simulink model "exercise02"  (R2022a)
settings: Solver=VariableStepAuto  StartTime=0.0  StopTime=10  RelTol=1e-3
settings Model: Creator=ac133867  LastModifiedBy=cunis
settings DebuggingCC: UnconnectedInputMsg=warning  UnconnectedOutputMsg=warning  UnconnectedLineMsg=warning
settings RTWCC: DLArmComputeVersion=19.05

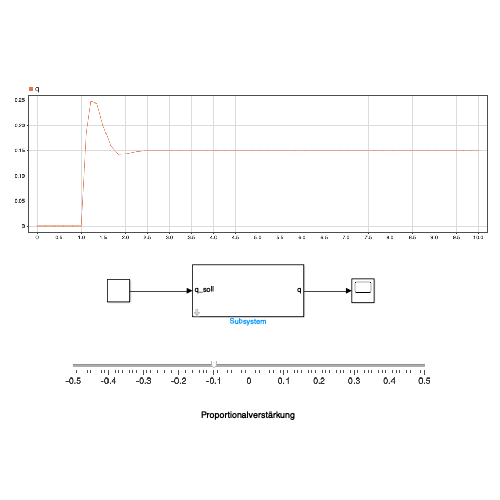
[thumbnail: Simulink's stored preview of the top-level diagram]
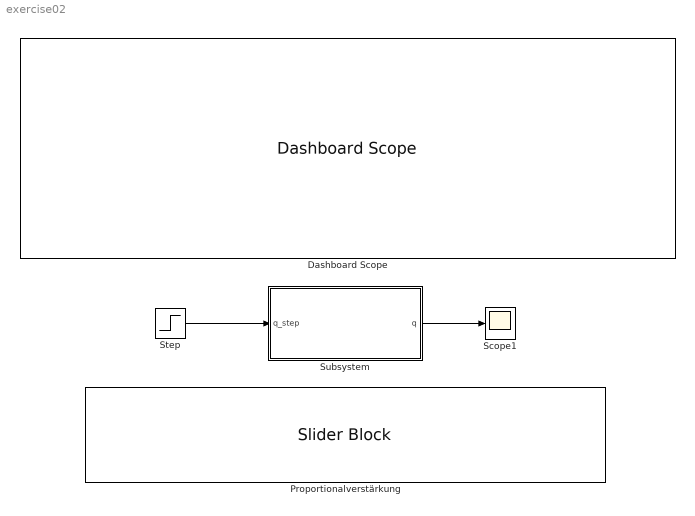
== system exercise02 ==
  Dashboard Scope : DashboardScope  Ymin=-0.5  Ymax=0.5
  Proportionalverstärkung : SliderBlock  LabelPosition=Hide  ScaleMin=-0.5  ScaleMax=0.5
  Scope1 : Scope
  Step : Step  SampleTime=0
  Subsystem : Subsystem
      mask Display:
      | port_label('input', 1, 'q_soll');
      | port_label('output', 1, 'q');
  wires:
  Subsystem/1(q) -> Scope1/1
  Step/1 -> Subsystem/1(q_step)

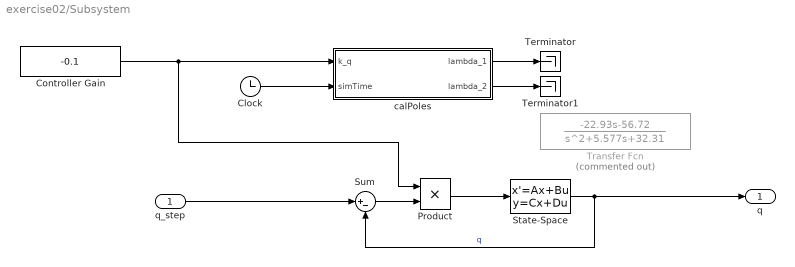
== system exercise02/Subsystem ==
  q_step : Inport
  Clock : Clock
  Controller Gain : Constant  Value=-0.1
  Product : Product
  State-Space : StateSpace  A=[-2.66012810859045,0.964626643293723;-25.4503792669483,-2.91714290772888]  B=[-0.168296921492111;-22.9341283239374]  C=[0 1]  D=0  InitialCondition=0
  Sum : Sum  Inputs=|+-
  Terminator : Terminator
  Terminator1 : Terminator
  Transfer Fcn : TransferFcn  Commented=on  Numerator=[-22.93 -56.72]  Denominator=[1 5.577 32.31]
  calPoles : MATLAB Function  TreatAsAtomicUnit=on
  q : Outport
  wires:
  q_step/1 -> Sum/1
  Controller Gain/1 -> Product/1, calPoles/1(k_q)
  State-Space/1 -> q/1, Sum/2  "q"
  Sum/1 -> Product/2
  Product/1 -> State-Space/1
  Clock/1 -> calPoles/2(simTime)
  calPoles/1(lambda_1) -> Terminator/1
  calPoles/2(lambda_2) -> Terminator1/1

== matlab function exercise02/Subsystem/calPoles ==
  data: k_q input; simTime input; lambda_1 output; lambda_2 output
function [lambda_1,lambda_2] = calcPoles(k_q,simTime)

% Anstellwinkelschwingung
A = [-2.66012810859045,0.964626643293723;-25.4503792669483,-2.91714290772888];
B = [-0.168296921492111;-22.9341283239374];


ZalphaV0   = A(1,1);
M_alpha   = A(2,1);
M_q       = A(2,2);

Z_etaV0   = B(1,1);
M_eta     = B(2,1);

% Eigenbewegung/ chara. Polynom
tmp = (M_eta*k_q - ZalphaV0 - M_q + Z_etaV0*k_q); % = 2*omega_0*zeta

omega_0sqrd = - M_alpha + M_q*ZalphaV0 + M_eta*k_q + M_alpha*Z_etaV0*k_q - M_q*Z_etaV0*k_q - M_eta*ZalphaV0*k_q;

omega_0 = sqrt(omega_0sqrd);
zeta    = tmp/(2*omega_0);

% Pole
lambda_1 = -zeta * omega_0 + omega_0 * sqrt(complex(zeta^2 - 1)); 
lambda_2 = -zeta * omega_0 - omega_0 * sqrt(complex(zeta^2 - 1)); 


% Plot only at the end
if simTime == 10
    close all
figure()
plot(lambda_1,'kx','LineWidth',1,'MarkerSize',10)
hold on
plot(lambda_2,'kx','LineWidth',1,'MarkerSize',10)
hold off
set(gca,'XLim',[-13 5]);
set(gca,'YLim',[-5.5 5.5]);
line([-13 5],[0 0],'Color','k')
line([0 0],[-5.5 5.5],'Color','k')
xlabel('Real Axis (1/seconds)')
ylabel('Imaginary Axis (1/seconds)')
grid on

else
end

end
